simulink model "test_matlabfunc"  (R2013b)
settings: Solver=ode45  StartTime=0.0  StopTime=40  RelTol=1e-3
values from neighbouring files (symbols this model uses):
  a = 1    [set_params_test_matlabfunc.m]    (also in test_sfunc_m.m = block.DialogPrm(1).Data)
  b = 2    [set_params_test_matlabfunc.m]    (also in test_sfunc_m.m = block.DialogPrm(2).Data)
  Ta = 0.1    [set_params_simulink_testfile.m]    (also in set_params_test_matlabfunc.m = 0.01)
  x0 = [0; 0]    [set_params_test_matlabfunc.m]    (also in test_sfunc_m.m = block.DialogPrm(3).Data)
settings Model: Creator=am  LastModifiedBy=zp
settings OptimizationCC: ExpressionDepthLimit=2147483647
settings DebuggingCC: StateNameClashWarn=warning

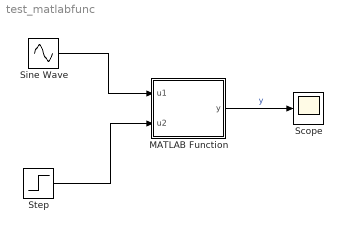
== system test_matlabfunc ==
  MATLAB Function : MATLAB Function  TreatAsAtomicUnit=on
  Scope : Scope
      settings: TimeRange=10  YMin=-0.1  YMax=0.6000000000000001
  Sine Wave : Sin  Frequency=0.25  SampleTime=0
  Step : Step  Time=10  After=0.1  SampleTime=0
  wires:
  MATLAB Function/1(y) -> Scope/1  "y"
  Sine Wave/1 -> MATLAB Function/1(u1)
  Step/1 -> MATLAB Function/2(u2)

== matlab function test_matlabfunc/MATLAB Function ==
  settings: updateMethod=DISCRETE  sampleTime=Ta
  data: u1 input; y output; b parameter; a parameter; x0 parameter; u2 input; Ta parameter
function y = fcn(u1, b, a, x0, u2, Ta)
%#codegen

% ------------------------------------------------------------------------
% Linken externer Matlab Funktionen
% ------------------------------------------------------------------------
coder.extrinsic('figure','plot');

% ------------------------------------------------------------------------
% Initialisierung der persistenten Variablen
% ------------------------------------------------------------------------

% Zustand
persistent x;
if(isempty(x))
    x = x0;
end

% Figure handle
persistent h;
if(isempty(h))
    h = figure;
end

% Counter
persistent count;
if(isempty(count))
    count = 1;
end

% ------------------------------------------------------------------------
% Programm
% ------------------------------------------------------------------------

% Aktuelle Ausgabe
y = [x(1);x(2);exp(x(1))*cosh(x(2))];

% Plotte Zustand im Phasenraum alle 10 Abtastwerte
if(count>=10)
    PlotXPhasenraum(x,h);
    count = 1;
end

% Loesung der ODE mittels explizitem Eulerverfahren
x = x + Ta*[-x(2) + sin(u1); a*x(1) + b*u2];
count = count + 1;
